simulink library "speedgoatlib"  (Simulink 7.6)
settings: Solver=ode45  StartTime=0.0  StopTime=10.0  RelTol=1e-3
undefined symbols (not defined in the file): m_XR17D15x, mmodemcontrol, standard
libraries: speedgoatlib x176, xpcseriallib x84, xpclib x4, simulink x4
(part 4 of 4)

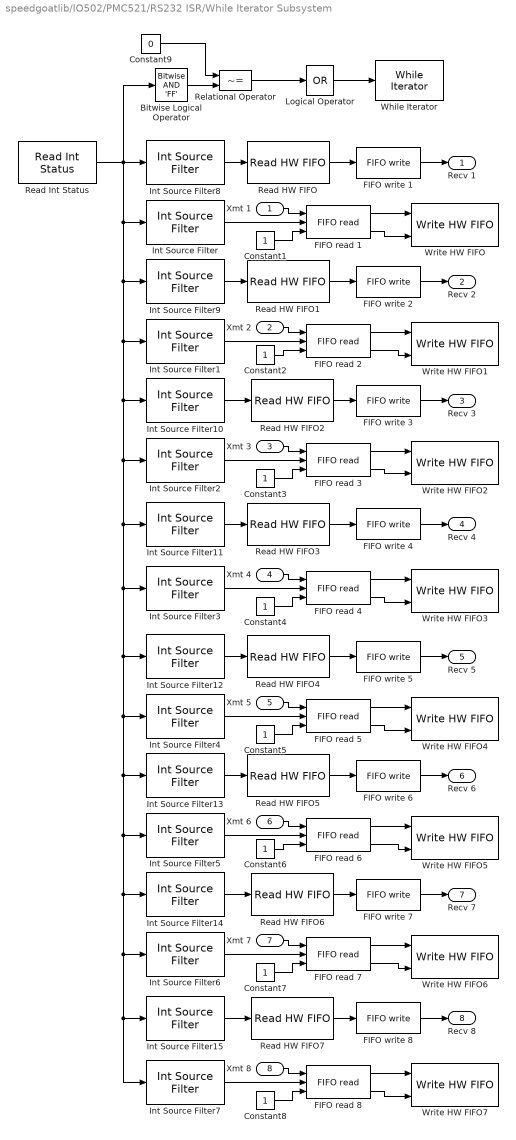
== system speedgoatlib/IO502/PMC521/RS232 ISR/While Iterator Subsystem ==
  Xmt 1 : Inport
  Xmt 2 : Inport  Port=2
  Xmt 3 : Inport  Port=3
  Xmt 4 : Inport  Port=4
  Xmt 5 : Inport  Port=5
  Xmt 6 : Inport  Port=6
  Xmt 7 : Inport  Port=7
  Xmt 8 : Inport  Port=8
  Bitwise Logical Operator : simulink/Logic and Bit Operations/Bitwise Operator  logicop=AND  UseBitMask=on  BitMask='FF'  BitMaskRealWorld=Stored Integer
  Constant{1..8} (8 alike) : Constant  OutDataTypeStr=uint32
  Constant9 : Constant  Value=0  OutDataTypeStr=uint32
  FIFO read {1..8} (8 alike) : xpcseriallib/FIFO read   maxsize=60  minsize=1  usedelimiter=off  delimiter=13  outputtype=count+32 bit uint  enable=on  enableout=on  sampletime=-1
  FIFO write 1 : xpcseriallib/FIFO write   size=1024  inputtype=count+32 bit uint  present=off  sampletime=-1  id=RCV channel 1, IRQ 5
  FIFO write 2 : xpcseriallib/FIFO write   size=1024  inputtype=count+32 bit uint  present=off  sampletime=-1  id=RCV channel 2, IRQ 5
  FIFO write 3 : xpcseriallib/FIFO write   size=1024  inputtype=count+32 bit uint  present=off  sampletime=-1  id=RCV channel 3, IRQ 5
  FIFO write 4 : xpcseriallib/FIFO write   size=1024  inputtype=count+32 bit uint  present=off  sampletime=-1  id=RCV channel 4, IRQ 5
  FIFO write 5 : xpcseriallib/FIFO write   size=1024  inputtype=count+32 bit uint  present=off  sampletime=-1  id=RCV channel 5, IRQ 5
  FIFO write 6 : xpcseriallib/FIFO write   size=1024  inputtype=count+32 bit uint  present=off  sampletime=-1  id=RCV channel 6, IRQ 5
  FIFO write 7 : xpcseriallib/FIFO write   size=1024  inputtype=count+32 bit uint  present=off  sampletime=-1  id=RCV channel 7, IRQ 5
  FIFO write 8 : xpcseriallib/FIFO write   size=1024  inputtype=count+32 bit uint  present=off  sampletime=-1  id=RCV channel 8, IRQ 5
  Int Source Filter : speedgoatlib/IO502/Acromag PMC521 Internal blocks/Int Source Filter  port=1  value=Transmitter empty
  Int Source Filter1 : speedgoatlib/IO502/Acromag PMC521 Internal blocks/Int Source Filter  port=2  value=Transmitter empty
  Int Source Filter10 : speedgoatlib/IO502/Acromag PMC521 Internal blocks/Int Source Filter  port=3  value=Receive data
  Int Source Filter11 : speedgoatlib/IO502/Acromag PMC521 Internal blocks/Int Source Filter  port=4  value=Receive data
  Int Source Filter12 : speedgoatlib/IO502/Acromag PMC521 Internal blocks/Int Source Filter  port=5  value=Receive data
  Int Source Filter13 : speedgoatlib/IO502/Acromag PMC521 Internal blocks/Int Source Filter  port=6  value=Receive data
  Int Source Filter14 : speedgoatlib/IO502/Acromag PMC521 Internal blocks/Int Source Filter  port=7  value=Receive data
  Int Source Filter15 : speedgoatlib/IO502/Acromag PMC521 Internal blocks/Int Source Filter  port=8  value=Receive data
  Int Source Filter2 : speedgoatlib/IO502/Acromag PMC521 Internal blocks/Int Source Filter  port=3  value=Transmitter empty
  Int Source Filter3 : speedgoatlib/IO502/Acromag PMC521 Internal blocks/Int Source Filter  port=4  value=Transmitter empty
  Int Source Filter4 : speedgoatlib/IO502/Acromag PMC521 Internal blocks/Int Source Filter  port=5  value=Transmitter empty
  Int Source Filter5 : speedgoatlib/IO502/Acromag PMC521 Internal blocks/Int Source Filter  port=6  value=Transmitter empty
  Int Source Filter6 : speedgoatlib/IO502/Acromag PMC521 Internal blocks/Int Source Filter  port=7  value=Transmitter empty
  Int Source Filter7 : speedgoatlib/IO502/Acromag PMC521 Internal blocks/Int Source Filter  port=8  value=Transmitter empty
  Int Source Filter8 : speedgoatlib/IO502/Acromag PMC521 Internal blocks/Int Source Filter  port=1  value=Receive data
  Int Source Filter9 : speedgoatlib/IO502/Acromag PMC521 Internal blocks/Int Source Filter  port=2  value=Receive data
  Logical Operator : Logic  Operator=OR  Inputs=1  AllPortsSameDT=off
  Read HW FIFO : speedgoatlib/IO502/Acromag PMC521 Internal blocks/Read HW FIFO  port=1  flush=on  slot=subslot
  Read HW FIFO1 : speedgoatlib/IO502/Acromag PMC521 Internal blocks/Read HW FIFO  port=2  flush=on  slot=subslot
  Read HW FIFO2 : speedgoatlib/IO502/Acromag PMC521 Internal blocks/Read HW FIFO  port=3  flush=on  slot=subslot
  Read HW FIFO3 : speedgoatlib/IO502/Acromag PMC521 Internal blocks/Read HW FIFO  port=4  flush=on  slot=subslot
  Read HW FIFO4 : speedgoatlib/IO502/Acromag PMC521 Internal blocks/Read HW FIFO  port=5  flush=on  slot=subslot
  Read HW FIFO5 : speedgoatlib/IO502/Acromag PMC521 Internal blocks/Read HW FIFO  port=6  flush=on  slot=subslot
  Read HW FIFO6 : speedgoatlib/IO502/Acromag PMC521 Internal blocks/Read HW FIFO  port=7  flush=on  slot=subslot
  Read HW FIFO7 : speedgoatlib/IO502/Acromag PMC521 Internal blocks/Read HW FIFO  port=8  flush=on  slot=subslot
  Read Int Status : speedgoatlib/IO502/Acromag PMC521 Internal blocks/Read Int Status  slot=subslot
  Relational Operator : RelationalOperator  Operator=~=
  While Iterator : WhileIterator  MaxIters=65  WhileBlockType=do-while
  Write HW FIFO : speedgoatlib/IO502/Acromag PMC521 Internal blocks/Write HW FIFO  port=1  slot=subslot
  Write HW FIFO1 : speedgoatlib/IO502/Acromag PMC521 Internal blocks/Write HW FIFO  port=2  slot=subslot
  Write HW FIFO2 : speedgoatlib/IO502/Acromag PMC521 Internal blocks/Write HW FIFO  port=3  slot=subslot
  Write HW FIFO3 : speedgoatlib/IO502/Acromag PMC521 Internal blocks/Write HW FIFO  port=4  slot=subslot
  Write HW FIFO4 : speedgoatlib/IO502/Acromag PMC521 Internal blocks/Write HW FIFO  port=5  slot=subslot
  Write HW FIFO5 : speedgoatlib/IO502/Acromag PMC521 Internal blocks/Write HW FIFO  port=6  slot=subslot
  Write HW FIFO6 : speedgoatlib/IO502/Acromag PMC521 Internal blocks/Write HW FIFO  port=7  slot=subslot
  Write HW FIFO7 : speedgoatlib/IO502/Acromag PMC521 Internal blocks/Write HW FIFO  port=8  slot=subslot
  Recv 1 : Outport
  Recv 2 : Outport  Port=2
  Recv 3 : Outport  Port=3
  Recv 4 : Outport  Port=4
  Recv 5 : Outport  Port=5
  Recv 6 : Outport  Port=6
  Recv 7 : Outport  Port=7
  Recv 8 : Outport  Port=8
  wires:
  Int Source Filter12/1 -> Read HW FIFO4/1
  FIFO write 5/1 -> Recv 5/1
  Read HW FIFO4/1 -> FIFO write 5/1
  Int Source Filter4/1 -> FIFO read 5/2
  Xmt 5/1 -> FIFO read 5/1
  Int Source Filter13/1 -> Read HW FIFO5/1
  FIFO write 6/1 -> Recv 6/1
  Read HW FIFO5/1 -> FIFO write 6/1
  Int Source Filter5/1 -> FIFO read 6/2
  Xmt 6/1 -> FIFO read 6/1
  FIFO read 6/1 -> Write HW FIFO5/1
  FIFO read 5/1 -> Write HW FIFO4/1
  FIFO read 5/2 -> Write HW FIFO4/2
  FIFO read 6/2 -> Write HW FIFO5/2
  Constant5/1 -> FIFO read 5/3
  Constant6/1 -> FIFO read 6/3
  Int Source Filter6/1 -> FIFO read 7/2
  Xmt 7/1 -> FIFO read 7/1
  FIFO read 7/1 -> Write HW FIFO6/1
  FIFO read 7/2 -> Write HW FIFO6/2
  Constant7/1 -> FIFO read 7/3
  Int Source Filter7/1 -> FIFO read 8/2
  Xmt 8/1 -> FIFO read 8/1
  FIFO read 8/1 -> Write HW FIFO7/1
  FIFO read 8/2 -> Write HW FIFO7/2
  Constant8/1 -> FIFO read 8/3
  Int Source Filter14/1 -> Read HW FIFO6/1
  Int Source Filter15/1 -> Read HW FIFO7/1
  FIFO write 7/1 -> Recv 7/1
  Read HW FIFO6/1 -> FIFO write 7/1
  FIFO write 8/1 -> Recv 8/1
  Read HW FIFO7/1 -> FIFO write 8/1
  Logical Operator/1 -> While Iterator/1
  Relational Operator/1 -> Logical Operator/1
  Bitwise Logical Operator/1 -> Relational Operator/2
  Constant9/1 -> Relational Operator/1
  Read Int Status/1 -> Int Source Filter8/1, Int Source Filter/1, Int Source Filter9/1, Int Source Filter1/1, Int Source Filter10/1, Int Source Filter2/1, Int Source Filter11/1, Int Source Filter3/1, Int Source Filter12/1, Int Source Filter4/1, Int Source Filter13/1, Int Source Filter5/1, Int Source Filter14/1, Int Source Filter6/1, Int Source Filter7/1, Int Source Filter15/1, Bitwise Logical Operator/1
  Int Source Filter8/1 -> Read HW FIFO/1
  FIFO write 1/1 -> Recv 1/1
  Read HW FIFO/1 -> FIFO write 1/1
  Int Source Filter/1 -> FIFO read 1/2
  Xmt 1/1 -> FIFO read 1/1
  Int Source Filter9/1 -> Read HW FIFO1/1
  FIFO write 2/1 -> Recv 2/1
  Read HW FIFO1/1 -> FIFO write 2/1
  Int Source Filter1/1 -> FIFO read 2/2
  Xmt 2/1 -> FIFO read 2/1
  FIFO read 2/1 -> Write HW FIFO1/1
  FIFO read 1/1 -> Write HW FIFO/1
  FIFO read 1/2 -> Write HW FIFO/2
  FIFO read 2/2 -> Write HW FIFO1/2
  Constant1/1 -> FIFO read 1/3
  Constant2/1 -> FIFO read 2/3
  Int Source Filter2/1 -> FIFO read 3/2
  Xmt 3/1 -> FIFO read 3/1
  FIFO read 3/1 -> Write HW FIFO2/1
  FIFO read 3/2 -> Write HW FIFO2/2
  Constant3/1 -> FIFO read 3/3
  Int Source Filter3/1 -> FIFO read 4/2
  Xmt 4/1 -> FIFO read 4/1
  FIFO read 4/1 -> Write HW FIFO3/1
  FIFO read 4/2 -> Write HW FIFO3/2
  Constant4/1 -> FIFO read 4/3
  Int Source Filter10/1 -> Read HW FIFO2/1
  Int Source Filter11/1 -> Read HW FIFO3/1
  FIFO write 3/1 -> Recv 3/1
  Read HW FIFO2/1 -> FIFO write 3/1
  FIFO write 4/1 -> Recv 4/1
  Read HW FIFO3/1 -> FIFO write 4/1

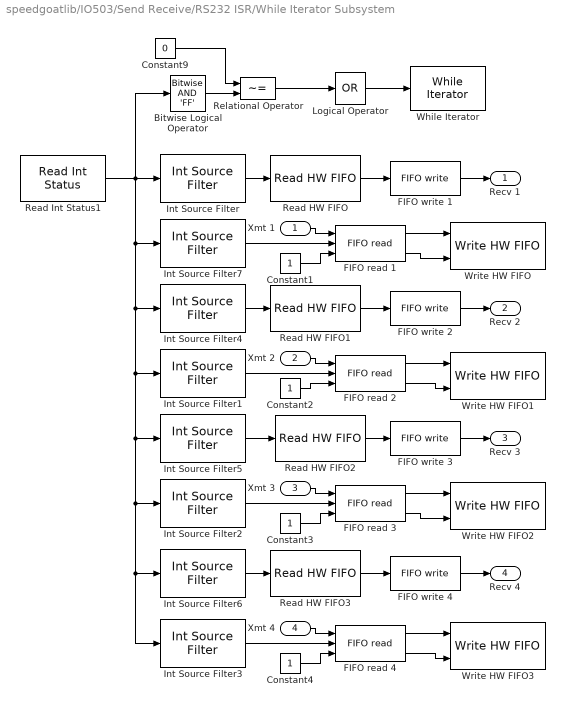
== system speedgoatlib/IO503/Send Receive/RS232 ISR/While Iterator Subsystem ==
  Xmt 1 : Inport
  Xmt 2 : Inport  Port=2
  Xmt 3 : Inport  Port=3
  Xmt 4 : Inport  Port=4
  Bitwise Logical Operator : simulink/Logic and Bit Operations/Bitwise Operator  logicop=AND  UseBitMask=on  BitMask='FF'  BitMaskRealWorld=Stored Integer
  Constant{1..4} (4 alike) : Constant  OutDataTypeStr=uint32
  Constant9 : Constant  Value=0  OutDataTypeStr=uint32
  FIFO read {1..4} (4 alike) : xpcseriallib/FIFO read   maxsize=60  minsize=1  usedelimiter=off  delimiter=13  outputtype=count+32 bit uint  enable=on  enableout=on  sampletime=-1
  FIFO write 1 : xpcseriallib/FIFO write   size=1024  inputtype=count+32 bit uint  present=off  sampletime=-1  id=RCV channel 1, IRQ 5
  FIFO write 2 : xpcseriallib/FIFO write   size=1024  inputtype=count+32 bit uint  present=off  sampletime=-1  id=RCV channel 2, IRQ 5
  FIFO write 3 : xpcseriallib/FIFO write   size=1024  inputtype=count+32 bit uint  present=off  sampletime=-1  id=RCV channel 3, IRQ 5
  FIFO write 4 : xpcseriallib/FIFO write   size=1024  inputtype=count+32 bit uint  present=off  sampletime=-1  id=RCV channel 4, IRQ 5
  Int Source Filter : speedgoatlib/IO503/Speedgoat IO503 Internal blocks/Int Source Filter  port=1  value=Receive data
  Int Source Filter1 : speedgoatlib/IO503/Speedgoat IO503 Internal blocks/Int Source Filter  port=2  value=Transmitter empty
  Int Source Filter2 : speedgoatlib/IO503/Speedgoat IO503 Internal blocks/Int Source Filter  port=3  value=Transmitter empty
  Int Source Filter3 : speedgoatlib/IO503/Speedgoat IO503 Internal blocks/Int Source Filter  port=4  value=Transmitter empty
  Int Source Filter4 : speedgoatlib/IO503/Speedgoat IO503 Internal blocks/Int Source Filter  port=2  value=Receive data
  Int Source Filter5 : speedgoatlib/IO503/Speedgoat IO503 Internal blocks/Int Source Filter  port=3  value=Receive data
  Int Source Filter6 : speedgoatlib/IO503/Speedgoat IO503 Internal blocks/Int Source Filter  port=4  value=Receive data
  Int Source Filter7 : speedgoatlib/IO503/Speedgoat IO503 Internal blocks/Int Source Filter  port=1  value=Transmitter empty
  Logical Operator : Logic  Operator=OR  Inputs=1  AllPortsSameDT=off
  Read HW FIFO : speedgoatlib/IO503/Speedgoat IO503 Internal blocks/Read HW FIFO  port=1  flush=on  slot=subslot
  Read HW FIFO1 : speedgoatlib/IO503/Speedgoat IO503 Internal blocks/Read HW FIFO  port=2  flush=on  slot=subslot
  Read HW FIFO2 : speedgoatlib/IO503/Speedgoat IO503 Internal blocks/Read HW FIFO  port=3  flush=on  slot=subslot
  Read HW FIFO3 : speedgoatlib/IO503/Speedgoat IO503 Internal blocks/Read HW FIFO  port=4  flush=on  slot=subslot
  Read Int Status1 : speedgoatlib/IO503/Speedgoat IO503 Internal blocks/Read Int Status  slot=subslot
  Relational Operator : RelationalOperator  Operator=~=
  While Iterator : WhileIterator  MaxIters=65  WhileBlockType=do-while
  Write HW FIFO : speedgoatlib/IO503/Speedgoat IO503 Internal blocks/Write HW FIFO  port=1  slot=subslot
  Write HW FIFO1 : speedgoatlib/IO503/Speedgoat IO503 Internal blocks/Write HW FIFO  port=2  slot=subslot
  Write HW FIFO2 : speedgoatlib/IO503/Speedgoat IO503 Internal blocks/Write HW FIFO  port=3  slot=subslot
  Write HW FIFO3 : speedgoatlib/IO503/Speedgoat IO503 Internal blocks/Write HW FIFO  port=4  slot=subslot
  Recv 1 : Outport
  Recv 2 : Outport  Port=2
  Recv 3 : Outport  Port=3
  Recv 4 : Outport  Port=4
  wires:
  Int Source Filter3/1 -> FIFO read 4/2
  Xmt 4/1 -> FIFO read 4/1
  FIFO read 4/1 -> Write HW FIFO3/1
  FIFO read 4/2 -> Write HW FIFO3/2
  Constant4/1 -> FIFO read 4/3
  Logical Operator/1 -> While Iterator/1
  Relational Operator/1 -> Logical Operator/1
  Bitwise Logical Operator/1 -> Relational Operator/2
  Constant9/1 -> Relational Operator/1
  Read Int Status1/1 -> Int Source Filter/1, Int Source Filter7/1, Int Source Filter4/1, Int Source Filter1/1, Int Source Filter5/1, Int Source Filter2/1, Int Source Filter3/1, Int Source Filter6/1, Bitwise Logical Operator/1
  Int Source Filter/1 -> Read HW FIFO/1
  FIFO write 1/1 -> Recv 1/1
  Read HW FIFO/1 -> FIFO write 1/1
  Int Source Filter7/1 -> FIFO read 1/2
  Xmt 1/1 -> FIFO read 1/1
  Int Source Filter4/1 -> Read HW FIFO1/1
  FIFO write 2/1 -> Recv 2/1
  Read HW FIFO1/1 -> FIFO write 2/1
  Int Source Filter1/1 -> FIFO read 2/2
  Xmt 2/1 -> FIFO read 2/1
  FIFO read 2/1 -> Write HW FIFO1/1
  FIFO read 1/1 -> Write HW FIFO/1
  FIFO read 1/2 -> Write HW FIFO/2
  FIFO read 2/2 -> Write HW FIFO1/2
  Constant1/1 -> FIFO read 1/3
  Constant2/1 -> FIFO read 2/3
  Int Source Filter2/1 -> FIFO read 3/2
  Xmt 3/1 -> FIFO read 3/1
  FIFO read 3/1 -> Write HW FIFO2/1
  FIFO read 3/2 -> Write HW FIFO2/2
  Constant3/1 -> FIFO read 3/3
  Int Source Filter5/1 -> Read HW FIFO2/1
  Int Source Filter6/1 -> Read HW FIFO3/1
  FIFO write 3/1 -> Recv 3/1
  Read HW FIFO2/1 -> FIFO write 3/1
  FIFO write 4/1 -> Recv 4/1
  Read HW FIFO3/1 -> FIFO write 4/1

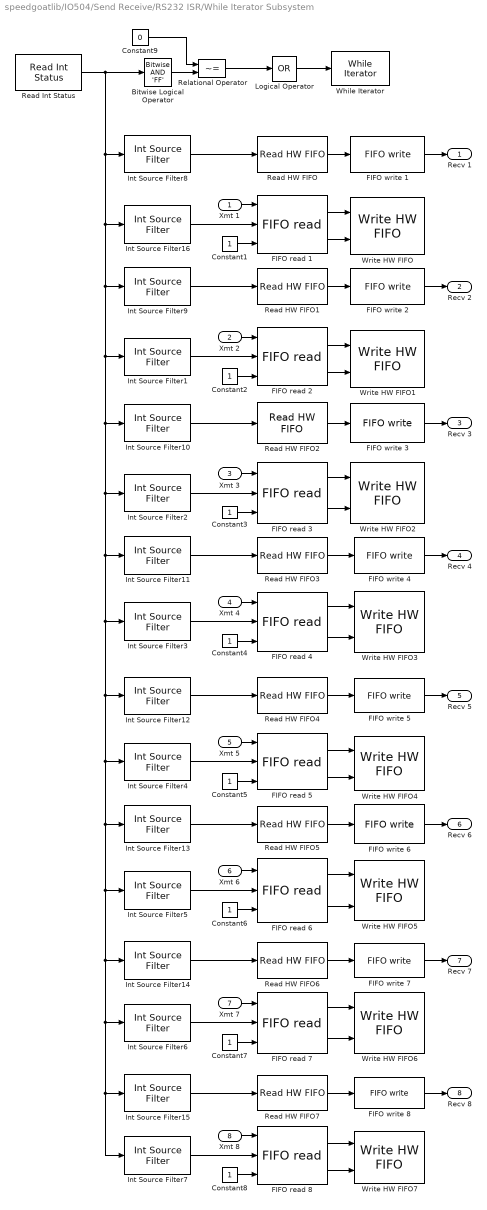
== system speedgoatlib/IO504/Send Receive/RS232 ISR/While Iterator Subsystem ==
  Xmt 1 : Inport
  Xmt 2 : Inport  Port=2
  Xmt 3 : Inport  Port=3
  Xmt 4 : Inport  Port=4
  Xmt 5 : Inport  Port=5
  Xmt 6 : Inport  Port=6
  Xmt 7 : Inport  Port=7
  Xmt 8 : Inport  Port=8
  Bitwise Logical Operator : simulink/Logic and Bit Operations/Bitwise Operator  logicop=AND  UseBitMask=on  BitMask='FF'  BitMaskRealWorld=Stored Integer
  Constant{1..8} (8 alike) : Constant  OutDataTypeStr=uint32
  Constant9 : Constant  Value=0  OutDataTypeStr=uint32
  FIFO read {1..8} (8 alike) : xpcseriallib/FIFO read   maxsize=60  minsize=1  usedelimiter=off  delimiter=13  outputtype=count+32 bit uint  enable=on  enableout=on  sampletime=-1
  FIFO write 1 : xpcseriallib/FIFO write   size=1024  inputtype=count+32 bit uint  present=off  sampletime=-1  id=RCV channel 1, IRQ 5
  FIFO write 2 : xpcseriallib/FIFO write   size=1024  inputtype=count+32 bit uint  present=off  sampletime=-1  id=RCV channel 2, IRQ 5
  FIFO write 3 : xpcseriallib/FIFO write   size=1024  inputtype=count+32 bit uint  present=off  sampletime=-1  id=RCV channel 3, IRQ 5
  FIFO write 4 : xpcseriallib/FIFO write   size=1024  inputtype=count+32 bit uint  present=off  sampletime=-1  id=RCV channel 4, IRQ 5
  FIFO write 5 : xpcseriallib/FIFO write   size=1024  inputtype=count+32 bit uint  present=off  sampletime=-1  id=RCV channel 5, IRQ 5
  FIFO write 6 : xpcseriallib/FIFO write   size=1024  inputtype=count+32 bit uint  present=off  sampletime=-1  id=RCV channel 6, IRQ 5
  FIFO write 7 : xpcseriallib/FIFO write   size=1024  inputtype=count+32 bit uint  present=off  sampletime=-1  id=RCV channel 7, IRQ 5
  FIFO write 8 : xpcseriallib/FIFO write   size=1024  inputtype=count+32 bit uint  present=off  sampletime=-1  id=RCV channel 8, IRQ 5
  Int Source Filter1 : speedgoatlib/IO504/Speedgoat IO504 Internal blocks/Int Source Filter  port=2  value=Transmitter empty
  Int Source Filter10 : speedgoatlib/IO504/Speedgoat IO504 Internal blocks/Int Source Filter  port=3  value=Receive data
  Int Source Filter11 : speedgoatlib/IO504/Speedgoat IO504 Internal blocks/Int Source Filter  port=4  value=Receive data
  Int Source Filter12 : speedgoatlib/IO504/Speedgoat IO504 Internal blocks/Int Source Filter  port=5  value=Receive data
  Int Source Filter13 : speedgoatlib/IO504/Speedgoat IO504 Internal blocks/Int Source Filter  port=6  value=Receive data
  Int Source Filter14 : speedgoatlib/IO504/Speedgoat IO504 Internal blocks/Int Source Filter  port=7  value=Receive data
  Int Source Filter15 : speedgoatlib/IO504/Speedgoat IO504 Internal blocks/Int Source Filter  port=8  value=Receive data
  Int Source Filter16 : speedgoatlib/IO504/Speedgoat IO504 Internal blocks/Int Source Filter  port=1  value=Transmitter empty
  Int Source Filter2 : speedgoatlib/IO504/Speedgoat IO504 Internal blocks/Int Source Filter  port=3  value=Transmitter empty
  Int Source Filter3 : speedgoatlib/IO504/Speedgoat IO504 Internal blocks/Int Source Filter  port=4  value=Transmitter empty
  Int Source Filter4 : speedgoatlib/IO504/Speedgoat IO504 Internal blocks/Int Source Filter  port=5  value=Transmitter empty
  Int Source Filter5 : speedgoatlib/IO504/Speedgoat IO504 Internal blocks/Int Source Filter  port=6  value=Transmitter empty
  Int Source Filter6 : speedgoatlib/IO504/Speedgoat IO504 Internal blocks/Int Source Filter  port=7  value=Transmitter empty
  Int Source Filter7 : speedgoatlib/IO504/Speedgoat IO504 Internal blocks/Int Source Filter  port=8  value=Transmitter empty
  Int Source Filter8 : speedgoatlib/IO504/Speedgoat IO504 Internal blocks/Int Source Filter  port=1  value=Receive data
  Int Source Filter9 : speedgoatlib/IO504/Speedgoat IO504 Internal blocks/Int Source Filter  port=2  value=Receive data
  Logical Operator : Logic  Operator=OR  Inputs=1  AllPortsSameDT=off
  Read HW FIFO : speedgoatlib/IO504/Speedgoat IO504 Internal blocks/Read HW FIFO  port=1  flush=on  slot=subslot
  Read HW FIFO1 : speedgoatlib/IO504/Speedgoat IO504 Internal blocks/Read HW FIFO  port=2  flush=on  slot=subslot
  Read HW FIFO2 : speedgoatlib/IO504/Speedgoat IO504 Internal blocks/Read HW FIFO  port=3  flush=on  slot=subslot
  Read HW FIFO3 : speedgoatlib/IO504/Speedgoat IO504 Internal blocks/Read HW FIFO  port=4  flush=on  slot=subslot
  Read HW FIFO4 : speedgoatlib/IO504/Speedgoat IO504 Internal blocks/Read HW FIFO  port=5  flush=on  slot=subslot
  Read HW FIFO5 : speedgoatlib/IO504/Speedgoat IO504 Internal blocks/Read HW FIFO  port=6  flush=on  slot=subslot
  Read HW FIFO6 : speedgoatlib/IO504/Speedgoat IO504 Internal blocks/Read HW FIFO  port=7  flush=on  slot=subslot
  Read HW FIFO7 : speedgoatlib/IO504/Speedgoat IO504 Internal blocks/Read HW FIFO  port=8  flush=on  slot=subslot
  Read Int Status : speedgoatlib/IO504/Speedgoat IO504 Internal blocks/Read Int Status  slot=subslot
  Relational Operator : RelationalOperator  Operator=~=
  While Iterator : WhileIterator  MaxIters=65  WhileBlockType=do-while
  Write HW FIFO : speedgoatlib/IO504/Speedgoat IO504 Internal blocks/Write HW FIFO  port=1  slot=subslot
  Write HW FIFO1 : speedgoatlib/IO504/Speedgoat IO504 Internal blocks/Write HW FIFO  port=2  slot=subslot
  Write HW FIFO2 : speedgoatlib/IO504/Speedgoat IO504 Internal blocks/Write HW FIFO  port=3  slot=subslot
  Write HW FIFO3 : speedgoatlib/IO504/Speedgoat IO504 Internal blocks/Write HW FIFO  port=4  slot=subslot
  Write HW FIFO4 : speedgoatlib/IO504/Speedgoat IO504 Internal blocks/Write HW FIFO  port=5  slot=subslot
  Write HW FIFO5 : speedgoatlib/IO504/Speedgoat IO504 Internal blocks/Write HW FIFO  port=6  slot=subslot
  Write HW FIFO6 : speedgoatlib/IO504/Speedgoat IO504 Internal blocks/Write HW FIFO  port=7  slot=subslot
  Write HW FIFO7 : speedgoatlib/IO504/Speedgoat IO504 Internal blocks/Write HW FIFO  port=8  slot=subslot
  Recv 1 : Outport
  Recv 2 : Outport  Port=2
  Recv 3 : Outport  Port=3
  Recv 4 : Outport  Port=4
  Recv 5 : Outport  Port=5
  Recv 6 : Outport  Port=6
  Recv 7 : Outport  Port=7
  Recv 8 : Outport  Port=8
  wires:
  Read HW FIFO3/1 -> FIFO write 4/1
  FIFO write 4/1 -> Recv 4/1
  Read HW FIFO2/1 -> FIFO write 3/1
  FIFO write 3/1 -> Recv 3/1
  Int Source Filter11/1 -> Read HW FIFO3/1
  Int Source Filter10/1 -> Read HW FIFO2/1
  Constant4/1 -> FIFO read 4/3
  FIFO read 4/2 -> Write HW FIFO3/2
  FIFO read 4/1 -> Write HW FIFO3/1
  Xmt 4/1 -> FIFO read 4/1
  Int Source Filter3/1 -> FIFO read 4/2
  Constant3/1 -> FIFO read 3/3
  FIFO read 3/2 -> Write HW FIFO2/2
  FIFO read 3/1 -> Write HW FIFO2/1
  Xmt 3/1 -> FIFO read 3/1
  Int Source Filter2/1 -> FIFO read 3/2
  Constant2/1 -> FIFO read 2/3
  Constant1/1 -> FIFO read 1/3
  FIFO read 2/2 -> Write HW FIFO1/2
  FIFO read 1/2 -> Write HW FIFO/2
  FIFO read 1/1 -> Write HW FIFO/1
  FIFO read 2/1 -> Write HW FIFO1/1
  Xmt 2/1 -> FIFO read 2/1
  Int Source Filter1/1 -> FIFO read 2/2
  Read HW FIFO1/1 -> FIFO write 2/1
  FIFO write 2/1 -> Recv 2/1
  Int Source Filter9/1 -> Read HW FIFO1/1
  Xmt 1/1 -> FIFO read 1/1
  Int Source Filter16/1 -> FIFO read 1/2
  Read HW FIFO/1 -> FIFO write 1/1
  FIFO write 1/1 -> Recv 1/1
  Int Source Filter8/1 -> Read HW FIFO/1
  Read Int Status/1 -> Int Source Filter8/1, Int Source Filter9/1, Int Source Filter1/1, Int Source Filter10/1, Int Source Filter2/1, Int Source Filter11/1, Int Source Filter3/1, Int Source Filter12/1, Int Source Filter4/1, Int Source Filter13/1, Int Source Filter14/1, Int Source Filter15/1, Int Source Filter7/1, Int Source Filter6/1, Int Source Filter5/1, Int Source Filter16/1, Bitwise Logical Operator/1
  Constant9/1 -> Relational Operator/1
  Bitwise Logical Operator/1 -> Relational Operator/2
  Relational Operator/1 -> Logical Operator/1
  Logical Operator/1 -> While Iterator/1
  Read HW FIFO7/1 -> FIFO write 8/1
  FIFO write 8/1 -> Recv 8/1
  Read HW FIFO6/1 -> FIFO write 7/1
  FIFO write 7/1 -> Recv 7/1
  Int Source Filter15/1 -> Read HW FIFO7/1
  Int Source Filter14/1 -> Read HW FIFO6/1
  Constant8/1 -> FIFO read 8/3
  FIFO read 8/2 -> Write HW FIFO7/2
  FIFO read 8/1 -> Write HW FIFO7/1
  Xmt 8/1 -> FIFO read 8/1
  Int Source Filter7/1 -> FIFO read 8/2
  Constant7/1 -> FIFO read 7/3
  FIFO read 7/2 -> Write HW FIFO6/2
  FIFO read 7/1 -> Write HW FIFO6/1
  Xmt 7/1 -> FIFO read 7/1
  Int Source Filter6/1 -> FIFO read 7/2
  Constant6/1 -> FIFO read 6/3
  Constant5/1 -> FIFO read 5/3
  FIFO read 6/2 -> Write HW FIFO5/2
  FIFO read 5/2 -> Write HW FIFO4/2
  FIFO read 5/1 -> Write HW FIFO4/1
  FIFO read 6/1 -> Write HW FIFO5/1
  Xmt 6/1 -> FIFO read 6/1
  Int Source Filter5/1 -> FIFO read 6/2
  Read HW FIFO5/1 -> FIFO write 6/1
  FIFO write 6/1 -> Recv 6/1
  Int Source Filter13/1 -> Read HW FIFO5/1
  Xmt 5/1 -> FIFO read 5/1
  Int Source Filter4/1 -> FIFO read 5/2
  Read HW FIFO4/1 -> FIFO write 5/1
  FIFO write 5/1 -> Recv 5/1
  Int Source Filter12/1 -> Read HW FIFO4/1
